simulink model "Model"  (R2020b)
settings: Solver=VariableStepAuto  StartTime=0.0  StopTime=10.0  RelTol=1e-3
settings Model: Creator=user  LastModifiedBy=user

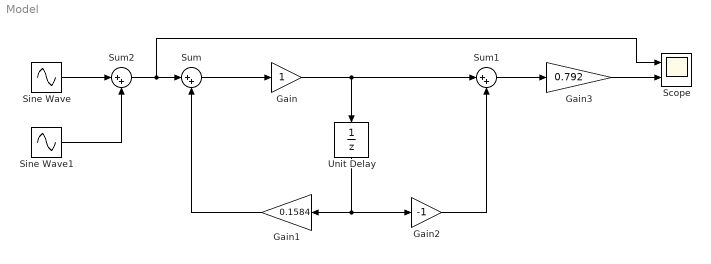
== system Model ==
  Gain : Gain
  Gain1 : Gain  Gain=0.1584
  Gain2 : Gain  Gain=-1
  Gain3 : Gain  Gain=0.792
  Scope : Scope  NumInputPorts=2
  Sine Wave : Sin  Amplitude=10  Frequency=10  SampleTime=0
  Sine Wave1 : Sin  Frequency=40000  SampleTime=0
  Sum : Sum  Inputs=|++
  Sum1 : Sum  Inputs=|++
  Sum2 : Sum  Inputs=|++
  Unit Delay : UnitDelay  SampleTime=-1  HasFrameUpgradeWarning=on
  wires:
  Sum/1 -> Gain/1
  Gain/1 -> Unit Delay/1, Sum1/1
  Unit Delay/1 -> Gain2/1, Gain1/1
  Gain1/1 -> Sum/2
  Gain2/1 -> Sum1/2
  Sum1/1 -> Gain3/1
  Gain3/1 -> Scope/2
  Sine Wave1/1 -> Sum2/2
  Sine Wave/1 -> Sum2/1
  Sum2/1 -> Scope/1, Sum/1
